simulink model "speedgoat_IO397_50k_all_io_2"  (R2019a)
settings: Solver=FixedStepDiscrete  StartTime=0.0  StopTime=inf  RelTol=1e-3  EnableMultiTasking=on
PreLoadFcn:
  | if ~exist('Ts', 'var')
  | Ts = 0.001;
  | end
  | if ~exist('FPGA_Frequency', 'var')
  | FPGA_Frequency = 75000000;
  | end
undefined symbols (not defined in the file): IO397
libraries: slrtlib x5, speedgoatlib_fpga_analog_io x2, simulink x2, speedgoatlib_fpga_dio x2, speedgoatlib_fpga x1, hdlsllib x1, speedgoatlib_fpga_inta x1
settings Model: Creator=ghetey  LastModifiedBy=sbeck
settings SolverCC: ConcurrentTasks=on  AutoInsertRateTranBlk=on
settings DataIOCC: SaveFormat=StructureWithTime
settings OptimizationCC: BlockReduction=off  OptimizeBlockIOStorage=off  BufferReuse=off  GlobalBufferReuse=off  ExpressionFolding=off  LocalBlockOutputs=off  OptimizeDataStoreBuffers=off  BusAssignmentInplaceUpdate=off
settings DebuggingCC: UnderspecifiedInitializationDetection=Classic  MergeDetectMultiDrivingBlocksExec=none  UnconnectedInputMsg=none  UnconnectedOutputMsg=none  UnconnectedLineMsg=none
settings HardwareCC: ProdBitPerPointer=32  ProdBitPerSizeT=32  ProdBitPerPtrDiffT=32  ProdLargestAtomicFloat=None  ProdWordSize=32  ProdLongLongMode=on  ProdHWDeviceType=Generic->32-bit x86 compatible
settings ModelReferenceCC: PropagateSignalLabelsOutOfModel=off
settings RTWCC: Description=Simulink Real-Time  SystemTargetFile=slrt.tlc  TemplateMakefile=slrt_default_tmf  CodeExecutionProfiling=on  RTWCompilerOptimization=on
settings SimulinkRealTimeCC: SupportVariableSizeSignals=on  PreserveStateflowLocalDataDimensions=off  RL32LogTETModifier=off  xPCConcurrentTasks=on

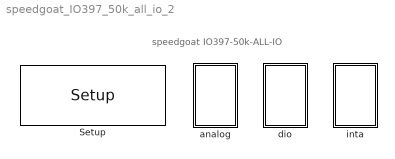
== system speedgoat_IO397_50k_all_io_2 ==
  note: speedgoat IO397-50k-ALL-IO
  Setup : speedgoatlib_fpga/Setup/Setup  board=IO397-50k  id=1  frontIO=None  rearIO=None  bitstreamFile=speedgoat_IO397_50k_all_io_2  rev=2.1  timestamp_string=dd/mm/yy hh:mm:ss  fpgaFreq=75 MHz  fpgaTick=13.3333 ns  ProgSpiFlash=off  ProgBPIFlash=off  pciSlot=-1  PullRPort0=pull-up 3.3V  VioPort0=3.3V  PullRPort1=pull-up 3.3V  VioPort1=3.3V  PullRPort2=pull-up 3.3V  VioPort2=3.3V  PullRPort3=pull-up 3.3V  VioPort3=3.3V  PullRPort4=pull-up 3.3V  VioPort4=3.3V  PullRPort5=pull-up 3.3V  VioPort5=3.3V  PullRPort6=pull-up 3.3V  VioPort6=3.3V  PullRPort15=pull-up 3.3V  PullRPort31=pull-up 3.3V  PullRPort47=pull-up 3.3V  PullRPort63=pull-up 3.3V
      settings: SourceProductName=Simulink Real-Time: Speedgoat Library
  analog : Subsystem
  dio : Subsystem
  inta : Subsystem

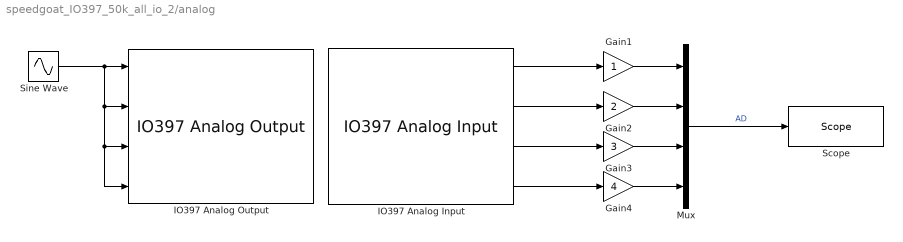
== system speedgoat_IO397_50k_all_io_2/analog ==
  Gain1 : Gain
  Gain2 : Gain  Gain=2
  Gain3 : Gain  Gain=3
  Gain4 : Gain  Gain=4
  IO397 Analog Input : speedgoatlib_fpga_analog_io/IO397 Analog Input  id=1  chan=[1:4]  range=+-5 V  trigger=Initiator  ts=0.001  pciSlot=-1  board=IO397-50k
      settings: SourceProductName=Simulink Real-Time: Speedgoat I/O Driver Library
  IO397 Analog Output : speedgoatlib_fpga_analog_io/IO397 Analog Output  id=1  chan=1:4  initVal=0  resetVal=0  ts=0.001  pciSlot=-1  board=IO397-50k  span=+-5 V
      settings: SourceProductName=Simulink Real-Time: Speedgoat I/O Driver Library
  Mux : Mux
  "Scope " : slrtlib/Displays and Logging/Scope   scopeno=1  scopetype=Target  autostart=on  viewmode=Graphical redraw  formatstr='%15.6f'  grid=on  ylimits=[0,0]  nosamples=250  noprepostsamples=0  interleave=1  triggermode=Signal triggering  triggersignal=1  trigsignalfromport=off  triggerlevel=0.5  triggerslope=Rising  triggerscope=1  triggersample=0  filename=data.dat  mode=Lazy  writesize=512  autorestart=off  dynamicfilemode=off  maxwritefilesize=512*1024^2
  Sine Wave : Sin  Frequency=2*pi*(1/Ts)/50  SampleTime=Ts
  wires:
  IO397 Analog Input/4 -> Gain4/1
  IO397 Analog Input/3 -> Gain3/1
  IO397 Analog Input/2 -> Gain2/1
  IO397 Analog Input/1 -> Gain1/1
  Gain4/1 -> Mux/4
  Gain3/1 -> Mux/3
  Gain2/1 -> Mux/2
  Gain1/1 -> Mux/1
  Sine Wave/1 -> IO397 Analog Output/1, IO397 Analog Output/3, IO397 Analog Output/4, IO397 Analog Output/2
  Mux/1 -> "Scope "/1  "AD"

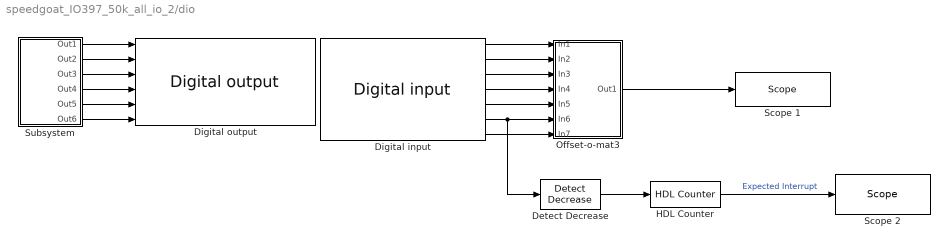
== system speedgoat_IO397_50k_all_io_2/dio ==
  Detect Decrease : simulink/Logic and Bit Operations/Detect Decrease  vinit=0.0  OutDataTypeStr=boolean
  Digital input : speedgoatlib_fpga_dio/Digital input  id=1  chan=[7:12,13]  ts=Ts  pciSlot=-1  board=IO397-50k  vectorizeOutput=off
      settings: SourceProductName=Simulink Real-Time: Speedgoat I/O Driver Library
  Digital output : speedgoatlib_fpga_dio/Digital output  id=1  chan=[1:6]  init=[0]  reset=[0]  vectorizeInput=off  ts=Ts  pciSlot=-1  board=IO397-50k
      settings: SourceProductName=Simulink Real-Time: Speedgoat I/O Driver Library
  HDL Counter : hdlsllib/Sources/HDL Counter  CountType=Free running  CountInit=0  CountStep=1  CountMax=25  CountFromType=Initial value  CountFrom=0  CountResetPort=off  CountLoadPort=off  CountEnbPort=on  CountDirPort=off  CountDataType=Unsigned  CountWordLen=32  CountFracLen=0  CountSampTime=1
      settings: SourceProductName=Simulink
  Offset-o-mat3 : Subsystem
  Scope 1 : slrtlib/Displays and Logging/Scope   scopeno=2  scopetype=Target  autostart=on  viewmode=Graphical redraw  formatstr='%15.6f'  grid=on  ylimits=[0,0]  nosamples=250  noprepostsamples=0  interleave=1  triggermode=FreeRun  triggersignal=1  trigsignalfromport=off  triggerlevel=0.0  triggerslope=Either  triggerscope=1  triggersample=0  filename=data.dat  mode=Lazy  writesize=512  autorestart=off  dynamicfilemode=off  maxwritefilesize=512*1024^2
  Scope 2 : slrtlib/Displays and Logging/Scope   scopeno=4  scopetype=Target  autostart=on  viewmode=Numerical  formatstr='%15.0f'  grid=on  ylimits=[0,0]  nosamples=3  noprepostsamples=0  interleave=1  triggermode=FreeRun  triggersignal=1  trigsignalfromport=off  triggerlevel=0.0  triggerslope=Either  triggerscope=1  triggersample=0  filename=data.dat  mode=Lazy  writesize=512  autorestart=off  dynamicfilemode=off  maxwritefilesize=512*1024^2
  Subsystem : Subsystem
  wires:
  Subsystem/4(Out4) -> Digital output/4
  Subsystem/3(Out3) -> Digital output/3
  Subsystem/2(Out2) -> Digital output/2
  Offset-o-mat3/1(Out1) -> Scope 1/1
  Subsystem/6(Out6) -> Digital output/6
  Subsystem/1(Out1) -> Digital output/1
  Subsystem/5(Out5) -> Digital output/5
  Digital input/1 -> Offset-o-mat3/1(In1)
  Digital input/2 -> Offset-o-mat3/2(In2)
  Digital input/3 -> Offset-o-mat3/3(In3)
  Digital input/4 -> Offset-o-mat3/4(In4)
  Digital input/5 -> Offset-o-mat3/5(In5)
  Digital input/6 -> Detect Decrease/1, Offset-o-mat3/6(In6)
  Digital input/7 -> Offset-o-mat3/7(In7)
  HDL Counter/1 -> Scope 2/1  "Expected Interrupt"
  Detect Decrease/1 -> HDL Counter/1

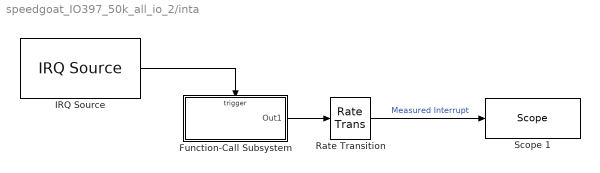
== system speedgoat_IO397_50k_all_io_2/inta ==
  Function-Call Subsystem : Subsystem  TreatAsAtomicUnit=on
  IRQ Source : slrtlib/Asynchronous Event/IRQ Source   irqNo=Auto (PCI only)  preempt=10  b_type=Speedgoat IO397-50k IntA  slot=-1  isrPrio=0
      settings: SourceProductName=Simulink Real-Time  SourceProductBaseCode=XP
  Rate Transition : RateTransition  Integrity=off
  Scope 1 : slrtlib/Displays and Logging/Scope   scopeno=3  scopetype=Target  autostart=on  viewmode=Numerical  formatstr='%15.0f'  grid=on  ylimits=[0,0]  nosamples=3  noprepostsamples=0  interleave=1  triggermode=FreeRun  triggersignal=1  trigsignalfromport=off  triggerlevel=0.0  triggerslope=Either  triggerscope=1  triggersample=0  filename=data.dat  mode=Lazy  writesize=512  autorestart=off  dynamicfilemode=off  maxwritefilesize=512*1024^2
  wires:
  Rate Transition/1 -> Scope 1/1  "Measured Interrupt"
  Function-Call Subsystem/1(Out1) -> Rate Transition/1
  IRQ Source/1 -> Function-Call Subsystem/Trigger

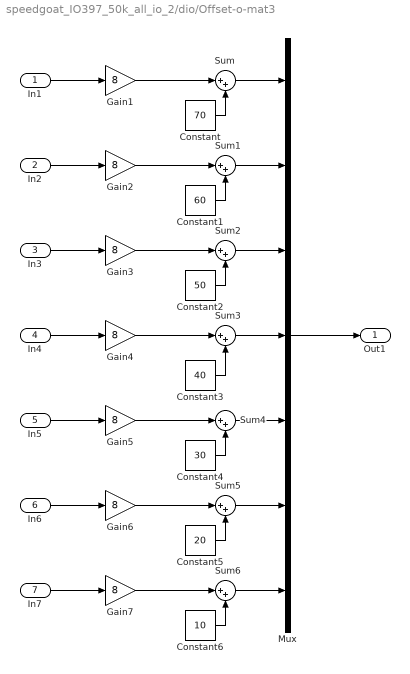
== system speedgoat_IO397_50k_all_io_2/dio/Offset-o-mat3 ==
  In1 : Inport
  In2 : Inport  Port=2
  In3 : Inport  Port=3
  In4 : Inport  Port=4
  In5 : Inport  Port=5
  In6 : Inport  Port=6
  In7 : Inport  Port=7
  Constant : Constant  Value=70
  Constant1 : Constant  Value=60
  Constant2 : Constant  Value=50
  Constant3 : Constant  Value=40
  Constant4 : Constant  Value=30
  Constant5 : Constant  Value=20
  Constant6 : Constant  Value=10
  Gain{1..7} (7 alike) : Gain  Gain=8
  Mux : Mux  Inputs=7
  Sum{,1..6} (7 alike) : Sum  Inputs=|++
  Out1 : Outport  VectorParamsAs1DForOutWhenUnconnected=off
  wires:
  Mux/1 -> Out1/1
  Constant/1 -> Sum/2
  In1/1 -> Gain1/1
  Sum/1 -> Mux/1
  Constant1/1 -> Sum1/2
  In2/1 -> Gain2/1
  Sum1/1 -> Mux/2
  Constant2/1 -> Sum2/2
  Sum2/1 -> Mux/3
  In3/1 -> Gain3/1
  In4/1 -> Gain4/1
  Gain1/1 -> Sum/1
  Gain2/1 -> Sum1/1
  Gain3/1 -> Sum2/1
  Constant3/1 -> Sum3/2
  Sum3/1 -> Mux/4
  Gain4/1 -> Sum3/1
  Constant4/1 -> Sum4/2
  In5/1 -> Gain5/1
  Sum4/1 -> Mux/5
  Constant5/1 -> Sum5/2
  In6/1 -> Gain6/1
  Sum5/1 -> Mux/6
  Gain5/1 -> Sum4/1
  Gain6/1 -> Sum5/1
  Gain7/1 -> Sum6/1
  Sum6/1 -> Mux/7
  In7/1 -> Gain7/1
  Constant6/1 -> Sum6/2

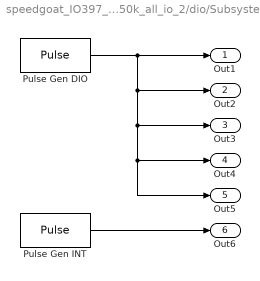
== system speedgoat_IO397_50k_all_io_2/dio/Subsystem ==
  Pulse Gen DIO : DiscretePulseGenerator  Period=20  PulseWidth=10  SampleTime=Ts  VectorParams1D=off
  Pulse Gen INT : DiscretePulseGenerator  SampleTime=Ts  VectorParams1D=off
  Out1 : Outport  VectorParamsAs1DForOutWhenUnconnected=off
  Out2 : Outport  Port=2  VectorParamsAs1DForOutWhenUnconnected=off
  Out3 : Outport  Port=3  VectorParamsAs1DForOutWhenUnconnected=off
  Out4 : Outport  Port=4  VectorParamsAs1DForOutWhenUnconnected=off
  Out5 : Outport  Port=5  VectorParamsAs1DForOutWhenUnconnected=off
  Out6 : Outport  Port=6  VectorParamsAs1DForOutWhenUnconnected=off
  wires:
  Pulse Gen DIO/1 -> Out1/1, Out5/1, Out4/1, Out3/1, Out2/1
  Pulse Gen INT/1 -> Out6/1

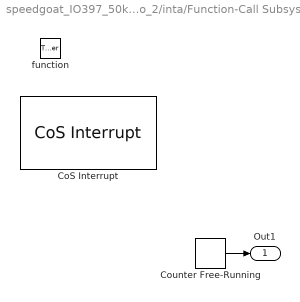
== system speedgoat_IO397_50k_all_io_2/inta/Function-Call Subsystem ==
  function : TriggerPort  TriggerType=function-call  VariantControl=Variant
  CoS Interrupt : speedgoatlib_fpga_inta/CoS Interrupt  id=1  debounce=10  delay=0  polarity=0  pciSlot=-1  ts=-1  board=IO397-50k
      settings: SourceProductName=Simulink Real-Time: Speedgoat I/O Driver Library
  Counter Free-Running : simulink/Sources/Counter Free-Running  NumBits=32  tsamp=-1
  Out1 : Outport  InitialOutput=[0]  VectorParamsAs1DForOutWhenUnconnected=off
  wires:
  Counter Free-Running/1 -> Out1/1
